simulink model "plot_f"  (R2023a)
settings: Solver=VariableStepAuto  StartTime=0.0  StopTime=15.0  RelTol=1e-3
values from neighbouring files (symbols this model uses):
  k = 100    [f.m]    (also in j.m)
  m = 200    [f.m]    (also in j.m)
settings Model: Creator=eriknymobohne  LastModifiedBy=eriknymobohne

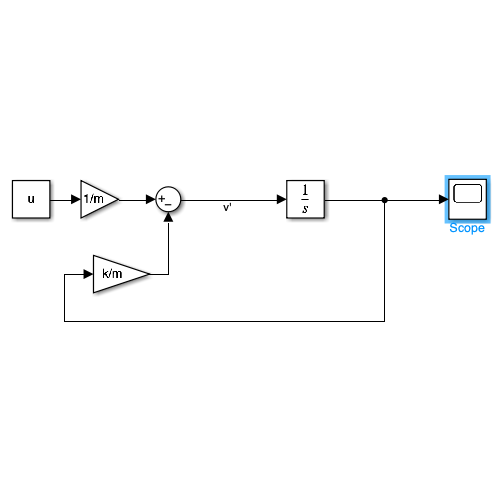
[thumbnail: Simulink's stored preview of the top-level diagram]
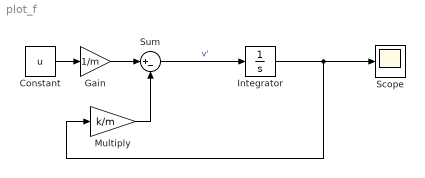
== system plot_f ==
  Constant : Constant  Value=u
  Gain : Gain  Gain=1/m
  Integrator : Integrator  InitialCondition=-5
  Multiply : Gain  Gain=k/m
  Scope : Scope
  Sum : Sum  Inputs=|+-
  wires:
  Integrator/1 -> Scope/1, Multiply/1
  Sum/1 -> Integrator/1  "v'"
  Multiply/1 -> Sum/2
  Constant/1 -> Gain/1
  Gain/1 -> Sum/1
